simulink model "Tricopter_Controlled"  (R2015a)
settings: Solver=ode3  SolverMode=SingleTasking  StartTime=0.0  StopTime=inf  FixedStep=T_sim  RelTol=1e-3
values from neighbouring files (symbols this model uses):
  A_l_max_x = sqrt( (A_z_max)^2  -  g^2  )    [Run3Copter.m]
  A_l_max_y = g*tand(15)    [Run3Copter.m]
  A_z_max = Max_Thrust*3/m    [Run3Copter.m]
  Alt_0 = input(' Give the initial altitude (m): ')    [Run3Copter.m]
  B_hover_4dof = [-0.192641491537 -0.295051706147 -72.3190840892 -0.00308714144823 24.9504828653 -1.18743631629 9.87469464114e-05 6.48783896558 -0.0529805907426 -0.000387203135788 0.131620058452 2.24065603044 ... (54 elements, 6x9)]    [Effectiv_matrices.mat]
  CG_0 = [0,0,0.02]'    [SetupComplete.m]
  epsilon = 0.01    [Run3Copter.m]
  eta_23 = deg2rad(-1.3)    [Run3Copter.m]
  g = 9.81    [SetupComplete.m]
  h = 0.08    [SetupComplete.m]
  h_M = 0.064    [SetupComplete.m]
  Hover_eta_23 = deg2rad(-1.3)    [Run3Copter.m]
  Hover_throtle_1 = 0.745    [Run3Copter.m]
  Hover_throtle_23 = Hover_throtle_1/cos(Hover_eta_23)    [Run3Copter.m]
  I_BAC_0 = [ Ix,0,Ixz;0,Iy,0;Ixz,0,Iz]    [SetupComplete.m]
  Initial_Omegas = Omega_hover    [Run3Copter.m]
  Initial_Torques = Torque_hover    [Run3Copter.m]
  Ix = 0.103    [SetupComplete.m]
  Iy = 0.147    [SetupComplete.m]
  Iz = 0.237    [SetupComplete.m]
  l = 0.345    [SetupComplete.m]
  l_arm = 0.264    [SetupComplete.m]
  latitude = 52.071118    [Run3Copter.m]
  longitude = -0.627404    [Run3Copter.m]
  m = 3.51    [SetupComplete.m]
  m_0 = 2.61    [SetupComplete.m]
  m_M = 0.300    (= 0.3)    [SetupComplete.m]
  Rotation_sign = [ 1,-1,-1]    [SetupComplete.m]
  T_ctrl = 0.02    [Run3Copter.m]
  T_sim = 0.01    [Run3Copter.m]
  throtle_1 = 0*0.745    (= 0)    [Run3Copter.m]
  throtle_23 = throtle_1/cos(eta_23)    [Run3Copter.m]
  v_i0 = sqrt( 1/3*m*g/(2*rho*pi*R^2)  )    [SetupComplete.m]
undefined symbols (not defined in the file or in its folder): DOWN_0, EAST_0, Newton, NORTH_0, P_0, Q_0, R_0, Raphson, U_0, V_0, W_0
libraries: XXCopter_Control x64, simulink_extras x17, simulink x11, XXCopter x8
(part 2 of 6)

== system Tricopter_Controlled/Sensors and filtering. No noise/Sensors and filtering. No noise ==
  state : Inport
  Bus Creator : BusCreator  Inputs=9
  Bus Selector2 : BusSelector  OutputSignals=X_e,V_b,V_e,omega_b,q,euler,A_s
  Current batrery level (V) : Constant  Value=14.8
  Demux : Demux  Outputs=3
  Gain{1..7} (7 alike) : Gain
  Gain8 : Gain  Gain=-1
  Terminator : Terminator
  Terminator1 : Terminator
  keep -pi/pi1 : Subsystem
  All_measures : Outport
  wires:
  keep -pi/pi1/1(out (rad)) -> Gain2/1
  Gain6/1 -> Bus Creator/1  "Pos meas (m)"
  Gain5/1 -> Bus Creator/6  "q_meas"
  Bus Selector2/5 -> Gain5/1  "<q>"
  Gain4/1 -> Bus Creator/4  "V_e_meas"
  Bus Selector2/3 -> Gain4/1  "<V_e>"
  Gain1/1 -> Bus Creator/8  "A_accel meas"
  Bus Selector2/7 -> Gain1/1  "<A_s>"
  Gain2/1 -> Bus Creator/7  "Euler meas (rad)"
  Demux/3 -> Gain8/1  "Alt meas (m)"
  Bus Creator/1 -> All_measures/1
  Gain3/1 -> Bus Creator/5  "omega_b meas (rad/s)"
  Gain7/1 -> Bus Creator/3  "V_b_meas"
  Bus Selector2/6 -> keep -pi/pi1/1(in (rad))  "<euler>"
  Bus Selector2/4 -> Gain3/1  "<omega_b>"
  Bus Selector2/2 -> Gain7/1  "<V_b>"
  Demux/2 -> Terminator1/1
  Demux/1 -> Terminator/1
  Gain8/1 -> Bus Creator/2  "Alt meas (m)"
  Bus Selector2/1 -> Demux/1, Gain6/1  "<X_e>"
  state/1 -> Bus Selector2/1
  Current batrery level (V)/1 -> Bus Creator/9  "Volt"

== system Tricopter_Controlled/Sensors and filtering. No noise/Sensors and filtering. Noise ==
  note: Basado en https://pixhawk.org/firmware/parameters#attitude_ekf_estimator
  state : Inport
  Add{1..5} (5 alike) : Sum  Inputs=++|
  Add6 : Sum  Inputs=|++
  Add7 : Sum  Inputs=|++
  Add8 : Sum  Inputs=|++
  Bus Creator : BusCreator  Inputs=9
  Bus Selector2 : BusSelector  OutputSignals=X_e,V_b,V_e,omega_b,q,euler,A_s
  Current batrery level (V) : Constant  Value=14.8
  Demux : Demux  Outputs=[2,1]
  Gain{1..7} (7 alike) : Gain
  Gain14 : Gain  Gain=[1;1;1]
  Gain8 : Gain  Gain=-1
  Mux : Mux  Inputs=[2,1]
  Uniform Random Number : UniformRandomNumber  Minimum=-0.5*[1;1]  Maximum=0.5*[1;1]  Seed=[1,4]  SampleTime=T_sim*2
  Uniform Random Number1 : UniformRandomNumber  Minimum=-0.1  Maximum=0.1  Seed=3  SampleTime=T_sim*2  VectorParams1D=off
  Uniform Random Number2 : UniformRandomNumber  Minimum=-0.05  Maximum=0.05  Seed=[4,5,8]  SampleTime=T_sim*2
  Uniform Random Number3 : UniformRandomNumber  Minimum=-0.05  Maximum=0.05  Seed=[4,5,8]  SampleTime=T_sim*2
  Uniform Random Number4 : UniformRandomNumber  Minimum=-deg2rad(0.01)  Maximum=deg2rad(0.01)  Seed=[47,6,80]  SampleTime=T_sim*2
  Uniform Random Number5 : UniformRandomNumber  Minimum=-deg2rad(0.1/360)  Maximum=deg2rad(0.1/360)  Seed=[4,78,8,2]  SampleTime=T_sim*2
  Uniform Random Number6 : UniformRandomNumber  Minimum=-deg2rad(0.1)  Maximum=deg2rad(0.1)  Seed=[40,50,80]  SampleTime=T_sim*2
  Uniform Random Number7 : UniformRandomNumber  Minimum=-0.01*9.81  Maximum=0.01*9.81  Seed=[4,5,8]  SampleTime=T_sim*2
  keep -pi/pi1 : Subsystem
  All_measures : Outport
  wires:
  Gain6/1 -> Bus Creator/1  "Pos meas (m)"
  Gain5/1 -> Bus Creator/6  "q_meas"
  Add2/1 -> Gain5/1
  Gain4/1 -> Bus Creator/4  "V_e_meas"
  Add8/1 -> Gain4/1
  Gain1/1 -> Bus Creator/8  "A_accel meas(m/s^2)"
  Gain2/1 -> Bus Creator/7  "Euler meas (rad)"
  Bus Creator/1 -> All_measures/1
  Gain3/1 -> Bus Creator/5  "omega_b meas (rad/s)"
  Gain7/1 -> Bus Creator/3  "V_b_meas"
  Bus Selector2/6 -> keep -pi/pi1/1(in (rad))  "<euler>"
  Add4/1 -> Gain3/1
  Add7/1 -> Gain7/1
  Gain8/1 -> Bus Creator/2  "Alt meas (m)"
  Bus Selector2/1 -> Demux/1  "<X_e>"
  state/1 -> Bus Selector2/1
  Bus Selector2/5 -> Add2/2  "<q>"
  Add1/1 -> Gain2/1
  keep -pi/pi1/1(out (rad)) -> Gain14/1
  Add3/1 -> Gain1/1
  Bus Selector2/7 -> Add3/2  "<A_s>"
  Bus Selector2/4 -> Add4/2  "<omega_b>"
  Demux/1 -> Add5/2
  Add5/1 -> Mux/1
  Add6/1 -> Gain8/1, Mux/2
  Demux/2 -> Add6/1
  Mux/1 -> Gain6/1
  Uniform Random Number1/1 -> Add6/2
  Bus Selector2/2 -> Add7/1  "<V_b>"
  Bus Selector2/3 -> Add8/1  "<V_e>"
  Uniform Random Number/1 -> Add5/1
  Uniform Random Number2/1 -> Add7/2
  Uniform Random Number3/1 -> Add8/2
  Uniform Random Number4/1 -> Add4/1
  Uniform Random Number5/1 -> Add2/1
  Gain14/1 -> Add1/2
  Uniform Random Number7/1 -> Add3/1
  Uniform Random Number6/1 -> Add1/1
  Current batrery level (V)/1 -> Bus Creator/9  "Volt"

== system Tricopter_Controlled/Signals reality/PWM resolution ==
  PWM_us in : Inport
  Quantizer : Quantizer  QuantizationInterval=5
  PWM_us out : Outport
  wires:
  PWM_us in/1 -> Quantizer/1
  Quantizer/1 -> PWM_us out/1

== system Tricopter_Controlled/Signals reality/PWM resolution1 ==
  PWM_us in : Inport
  Quantizer : Quantizer  QuantizationInterval=5
  PWM_us out : Outport
  wires:
  Quantizer/1 -> PWM_us out/1
  PWM_us in/1 -> Quantizer/1

== system Tricopter_Controlled/Signals reality/Re-Build Signals servos ==
  note: Control input
      | Rango
      | Direccion rot/Dir servos
      | Rango del servo
      |
      | eta_1 (rad) (Pan arm 1)
      | -165,165
      | -1
      | 330: -165,165
      |
      | gamma_1 (rad) (Tilt arm 1)
      | -90,15
      | -1
      | 180:-90,90 ó 330: -165,165
      |
      | eta_2 (rad) (Pan arm 2)
      | -165,165
      | -1
      | 330: -165,165
      |
      | gamma_2 (rad) (Tilt arm 2)
      | -15,90
      | 1
      | 180:-90,90
      |
      | eta_3 (rad) (Pan arm 3)
      | -165,165
      | 1
      | 330:-165,165
      |
      | gamma_3 (rad) (Tilt arm 3)
      | -90,15
      | -1
      | 180:-90,90
  PWM_us servos in : Inport
  Demux : Demux  Outputs=6
  Mux : Mux  Inputs=6
  PWM2signal : XXCopter_Control/PWM2signal  c=2100  a=900  d=deg2rad(90)  b=-deg2rad(90)
  PWM2signal1 : XXCopter_Control/PWM2signal  c=2100  a=900  d=deg2rad(165)  b=-deg2rad(165)
  PWM2signal2 : XXCopter_Control/PWM2signal  c=2100  a=900  d=deg2rad(90)  b=-deg2rad(90)
  PWM2signal3 : XXCopter_Control/PWM2signal  c=2100  a=900  d=deg2rad(90)  b=-deg2rad(90)
  PWM2signal4 : XXCopter_Control/PWM2signal  c=2100  a=900  d=deg2rad(165)  b=-deg2rad(165)
  PWM2signal5 : XXCopter_Control/PWM2signal  c=2100  a=900  d=deg2rad(165)  b=-deg2rad(165)
  Unary Minus{,1..3} (4 alike) : UnaryMinus
  signals out : Outport
  wires:
  PWM_us servos in/1 -> Demux/1
  Demux/6 -> PWM2signal3/1
  Demux/5 -> PWM2signal5/1
  Demux/4 -> PWM2signal2/1
  Demux/3 -> PWM2signal4/1
  Demux/2 -> PWM2signal/1
  Demux/1 -> PWM2signal1/1
  PWM2signal1/1 -> Unary Minus/1
  PWM2signal/1 -> Unary Minus1/1
  PWM2signal4/1 -> Unary Minus2/1
  PWM2signal2/1 -> Mux/4
  PWM2signal5/1 -> Mux/5
  PWM2signal3/1 -> Unary Minus3/1
  Mux/1 -> signals out/1
  Unary Minus/1 -> Mux/1
  Unary Minus1/1 -> Mux/2
  Unary Minus2/1 -> Mux/3
  Unary Minus3/1 -> Mux/6

== system Tricopter_Controlled/TriCopter FCS/Interface out ==
  In1 : Inport
  In2 : Inport  Port=2
  In3 : Inport  Port=3
  In4 : Inport  Port=4
  In5 : Inport  Port=5
  In6 : Inport  Port=6
  In7 : Inport  Port=7
  In8 : Inport  Port=8
  In9 : Inport  Port=9
  Mux : Mux  Inputs=3
  Mux1 : Mux  Inputs=6
  Out1 : Outport
  Out2 : Outport  Port=2
  wires:
  Mux/1 -> Out1/1
  In1/1 -> Mux/1
  In4/1 -> Mux/2
  In7/1 -> Mux/3
  In2/1 -> Mux1/1
  In3/1 -> Mux1/2
  In5/1 -> Mux1/3
  In6/1 -> Mux1/4
  In8/1 -> Mux1/5
  In9/1 -> Mux1/6
  Mux1/1 -> Out2/1

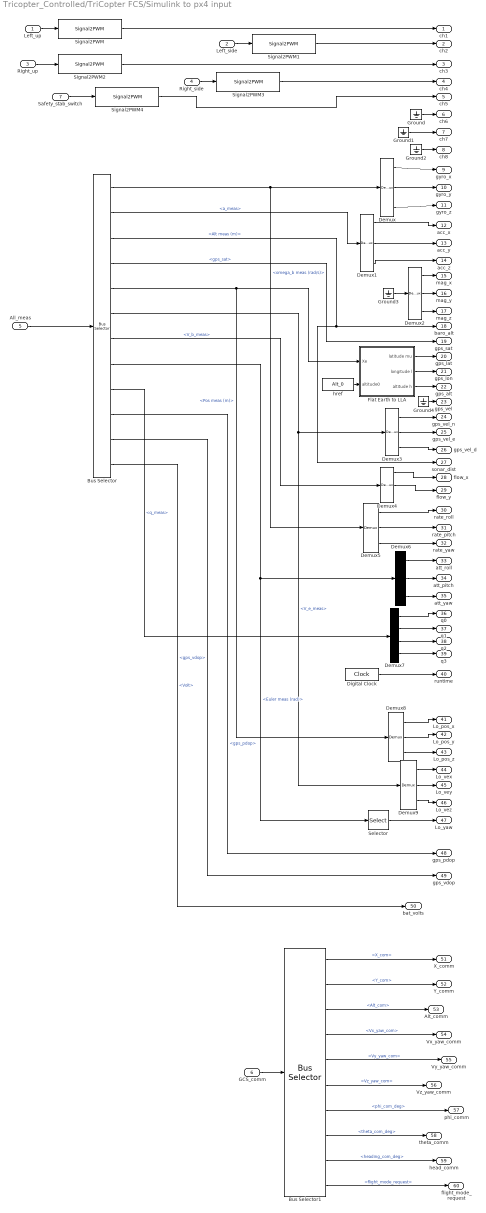
== system Tricopter_Controlled/TriCopter FCS/Simulink to px4 input ==
  Left_up : Inport
  Left_side : Inport  Port=2
  Right_up : Inport  Port=3
  Right_side : Inport  Port=4
  All_meas : Inport  Port=5
  GCS_comm : Inport  Port=6
  Safety_stab_switch : Inport  Port=7
  Bus Selector : BusSelector  OutputSignals=Meas.omega_b meas (rad/s),Params.a_meas,Meas.Alt meas (m),Params.gps_sat,Meas.Pos meas (m),Meas.V_e_meas,Meas.V_b_meas,Meas.Euler meas (rad),Meas.q_meas,Params.gps_pdop,Params.gps_vdop,Meas.Volt
  Bus Selector1 : BusSelector  OutputSignals=X_com,Y_com,Alt_com,Vx_yaw_com,Vy_yaw_com,Vz_yaw_com,phi_com_deg,theta_com_deg,heading_com_deg,flight_mode_request
  Demux{,1..6,8..9} (9 alike) : Demux  Outputs=3
  Demux7 : Demux
  Digital Clock : DigitalClock  SampleTime=T_ctrl
  Flat Earth to LLA : Subsystem
  Ground{,1..4} (5 alike) : Ground
  Selector : Selector  InputPortWidth=3  Indices=3
  Signal2PWM{,1..3} (4 alike) : XXCopter_Control/Signal2PWM  b=1  d=-1  a=1800  c=1200
  Signal2PWM4 : XXCopter_Control/Signal2PWM  b=1  d=0  a=1800  c=1200
  href : Constant  Value=Alt_0  VectorParams1D=off
  ch1 : Outport
  ch2 : Outport  Port=2
  ch3 : Outport  Port=3
  ch4 : Outport  Port=4
  ch5 : Outport  Port=5
  ch6 : Outport  Port=6
  ch7 : Outport  Port=7
  ch8 : Outport  Port=8
  gyro_x : Outport  Port=9
  gyro_y : Outport  Port=10
  gyro_z : Outport  Port=11
  acc_x : Outport  Port=12
  acc_y : Outport  Port=13
  acc_z : Outport  Port=14
  mag_x : Outport  Port=15
  mag_y : Outport  Port=16
  mag_z : Outport  Port=17
  baro_alt : Outport  Port=18
  gps_sat : Outport  Port=19
  gps_lat : Outport  Port=20
  gps_lon : Outport  Port=21
  gps_alt : Outport  Port=22
  gps_vel : Outport  Port=23
  gps_vel_n : Outport  Port=24
  gps_vel_e : Outport  Port=25
  gps_vel_d : Outport  Port=26
  sonar_dist : Outport  Port=27
  flow_x : Outport  Port=28
  flow_y : Outport  Port=29
  rate_roll : Outport  Port=30
  rate_pitch : Outport  Port=31
  rate_yaw : Outport  Port=32
  att_roll : Outport  Port=33
  att_pitch : Outport  Port=34
  att_yaw : Outport  Port=35
  q0 : Outport  Port=36
  q1 : Outport  Port=37
  q2 : Outport  Port=38
  q3 : Outport  Port=39
  runtime : Outport  Port=40
  Lo_pos_x : Outport  Port=41
  Lo_pos_y : Outport  Port=42
  Lo_pos_z : Outport  Port=43
  Lo_vex : Outport  Port=44
  Lo_vey : Outport  Port=45
  Lo_vez : Outport  Port=46
  Lo_yaw : Outport  Port=47
  gps_pdop : Outport  Port=48
  gps_vdop : Outport  Port=49
  bat_volts : Outport  Port=50
  X_comm : Outport  Port=51
  Y_comm : Outport  Port=52
  Alt_comm : Outport  Port=53
  Vx_yaw_comm : Outport  Port=54
  Vy_yaw_comm : Outport  Port=55
  Vz_yaw_comm : Outport  Port=56
  phi_comm : Outport  Port=57
  theta_comm : Outport  Port=58
  head_comm : Outport  Port=59
  flight_mode_request : Outport  Port=60
  wires:
  Left_up/1 -> Signal2PWM/1
  Left_side/1 -> Signal2PWM1/1
  Right_up/1 -> Signal2PWM2/1
  Right_side/1 -> Signal2PWM3/1
  Safety_stab_switch/1 -> Signal2PWM4/1
  Ground/1 -> ch6/1
  Ground1/1 -> ch7/1
  Ground2/1 -> ch8/1
  All_meas/1 -> Bus Selector/1
  href/1 -> Flat Earth to LLA/2(altitude0)
  Demux/1 -> gyro_x/1
  Demux/2 -> gyro_y/1
  Demux/3 -> gyro_z/1
  Bus Selector/1 -> Demux5/1, Demux/1  "<omega_b meas (rad/s)>"
  Demux1/1 -> acc_x/1
  Demux1/2 -> acc_y/1
  Demux1/3 -> acc_z/1
  Bus Selector/2 -> Demux1/1  "<a_meas>"
  Ground3/1 -> Demux2/1
  Demux2/1 -> mag_x/1
  Demux2/2 -> mag_y/1
  Demux2/3 -> mag_z/1
  Bus Selector/3 -> baro_alt/1, sonar_dist/1  "<Alt meas (m)>"
  Bus Selector/4 -> gps_sat/1  "<gps_sat>"
  Flat Earth to LLA/1(latitude mu) -> gps_lat/1
  Flat Earth to LLA/2(longitude l) -> gps_lon/1
  Flat Earth to LLA/3(altitude h) -> gps_alt/1
  Bus Selector/5 -> Flat Earth to LLA/1(Xe), Demux8/1  "<Pos meas (m)>"
  Ground4/1 -> gps_vel/1
  Demux3/1 -> gps_vel_n/1
  Demux3/3 -> gps_vel_d/1
  Bus Selector/6 -> Demux9/1, Demux3/1  "<V_e_meas>"
  Demux3/2 -> gps_vel_e/1
  Bus Selector/7 -> Demux4/1  "<V_b_meas>"
  Demux4/2 -> flow_y/1
  Demux4/1 -> flow_x/1
  Demux5/1 -> rate_roll/1
  Demux5/2 -> rate_pitch/1
  Demux5/3 -> rate_yaw/1
  Demux6/1 -> att_roll/1
  Demux6/2 -> att_pitch/1
  Demux6/3 -> att_yaw/1
  Bus Selector/8 -> Selector/1, Demux6/1  "<Euler meas (rad)>"
  Demux7/1 -> q0/1
  Demux7/2 -> q1/1
  Demux7/3 -> q2/1
  Demux7/4 -> q3/1
  Bus Selector/9 -> Demux7/1  "<q_meas>"
  Demux8/1 -> Lo_pos_x/1
  Demux8/2 -> Lo_pos_y/1
  Demux8/3 -> Lo_pos_z/1
  Demux9/1 -> Lo_vex/1
  Demux9/2 -> Lo_vey/1
  Demux9/3 -> Lo_vez/1
  Selector/1 -> Lo_yaw/1
  Bus Selector/10 -> gps_pdop/1  "<gps_pdop>"
  Bus Selector/11 -> gps_vdop/1  "<gps_vdop>"
  Bus Selector/12 -> bat_volts/1  "<Volt>"
  GCS_comm/1 -> Bus Selector1/1
  Bus Selector1/1 -> X_comm/1  "<X_com>"
  Bus Selector1/2 -> Y_comm/1  "<Y_com>"
  Bus Selector1/3 -> Alt_comm/1  "<Alt_com>"
  Bus Selector1/4 -> Vx_yaw_comm/1  "<Vx_yaw_com>"
  Bus Selector1/5 -> Vy_yaw_comm/1  "<Vy_yaw_com>"
  Bus Selector1/6 -> Vz_yaw_comm/1  "<Vz_yaw_com>"
  Bus Selector1/7 -> phi_comm/1  "<phi_com_deg>"
  Bus Selector1/8 -> theta_comm/1  "<theta_com_deg>"
  Bus Selector1/9 -> head_comm/1  "<heading_com_deg>"
  Bus Selector1/10 -> flight_mode_request/1  "<flight_mode_request>"
  Signal2PWM/1 -> ch1/1
  Signal2PWM1/1 -> ch2/1
  Signal2PWM2/1 -> ch3/1
  Signal2PWM3/1 -> ch4/1
  Signal2PWM4/1 -> ch5/1
  Digital Clock/1 -> runtime/1

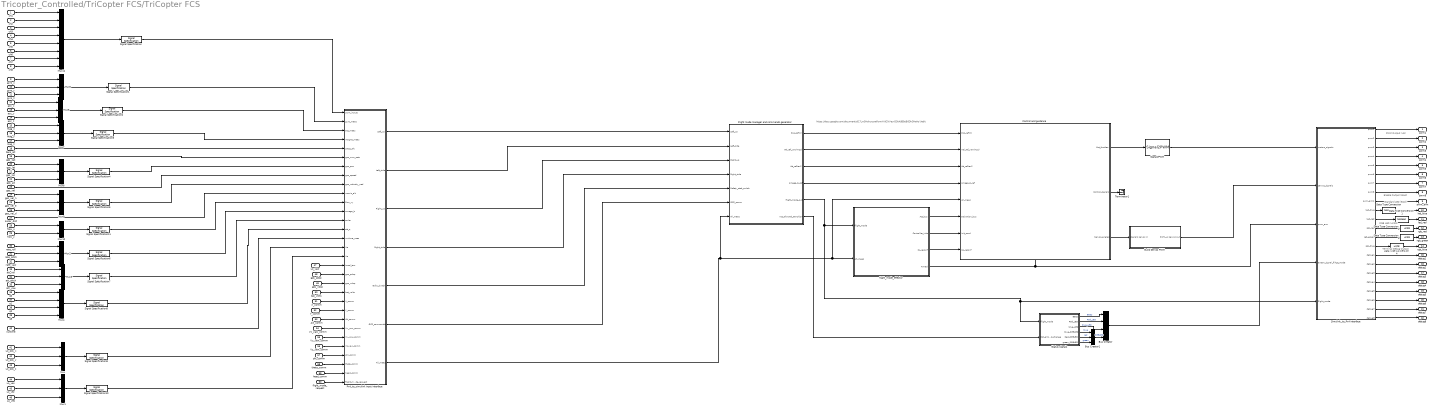
== system Tricopter_Controlled/TriCopter FCS/TriCopter FCS ==
  note: https://docs.google.com/document/d/17Lw5HdxcxpxePsmAYdCNVeyrDDt4j9EbtB6DkGHaHsY/edit
  note: Terminal Debug Output
  note: RGB LED (uint8)
  note: Standard LED (Bool)
  note: PWM Output (uS)
  note: Enable Output (Bool)
  ch1 : Inport  PortDimensions=[1,1]  SampleTime=T_ctrl
  ch2 : Inport  Port=2  PortDimensions=[1,1]  SampleTime=T_ctrl
  ch3 : Inport  Port=3  PortDimensions=[1,1]  SampleTime=T_ctrl
  ch4 : Inport  Port=4  PortDimensions=[1,1]  SampleTime=T_ctrl
  ch5 : Inport  Port=5  PortDimensions=[1,1]  SampleTime=T_ctrl
  ch6 : Inport  Port=6  PortDimensions=[1,1]  SampleTime=T_ctrl
  ch7 : Inport  Port=7  PortDimensions=[1,1]  SampleTime=T_ctrl
  ch8 : Inport  Port=8  PortDimensions=[1,1]  SampleTime=T_ctrl
  gyro_x : Inport  Port=9  PortDimensions=[1,1]  SampleTime=T_ctrl
  gyro_y : Inport  Port=10  PortDimensions=[1,1]  SampleTime=T_ctrl
  gyro_z : Inport  Port=11  PortDimensions=[1,1]  SampleTime=T_ctrl
  acc_x : Inport  Port=12  PortDimensions=[1,1]  SampleTime=T_ctrl
  acc_y : Inport  Port=13  PortDimensions=[1,1]  SampleTime=T_ctrl
  acc_z : Inport  Port=14  PortDimensions=[1,1]  SampleTime=T_ctrl
  mag_x : Inport  Port=15  PortDimensions=[1,1]  SampleTime=T_ctrl
  mag_y : Inport  Port=16  PortDimensions=[1,1]  SampleTime=T_ctrl
  mag_z : Inport  Port=17  PortDimensions=[1,1]  SampleTime=T_ctrl
  baro_alt : Inport  Port=18  PortDimensions=[1,1]  SampleTime=T_ctrl
  gps_sat : Inport  Port=19  PortDimensions=[1,1]  SampleTime=T_ctrl
  gps_lat : Inport  Port=20  PortDimensions=[1,1]  SampleTime=T_ctrl
  gps_lon : Inport  Port=21  PortDimensions=[1,1]  SampleTime=T_ctrl
  gps_alt : Inport  Port=22  PortDimensions=[1,1]  SampleTime=T_ctrl
  gps_vel : Inport  Port=23  PortDimensions=[1,1]  SampleTime=T_ctrl
  gps_vel_n : Inport  Port=24  PortDimensions=[1,1]  SampleTime=T_ctrl
  gps_vel_e : Inport  Port=25  PortDimensions=[1,1]  SampleTime=T_ctrl
  gps_vel_d : Inport  Port=26  PortDimensions=[1,1]  SampleTime=T_ctrl
  sonar_dist : Inport  Port=27  PortDimensions=[1,1]  SampleTime=T_ctrl
  flow_x : Inport  Port=28  PortDimensions=[1,1]  SampleTime=T_ctrl
  flow_y : Inport  Port=29  PortDimensions=[1,1]  SampleTime=T_ctrl
  rate_roll : Inport  Port=30  PortDimensions=[1,1]  SampleTime=T_ctrl
  rate_pitch : Inport  Port=31  PortDimensions=[1,1]  SampleTime=T_ctrl
  rate_yaw : Inport  Port=32  PortDimensions=[1,1]  SampleTime=T_ctrl
  att_roll : Inport  Port=33  PortDimensions=[1,1]  SampleTime=T_ctrl
  att_pitch : Inport  Port=34  PortDimensions=[1,1]  SampleTime=T_ctrl
  att_yaw : Inport  Port=35  PortDimensions=[1,1]  SampleTime=T_ctrl
  q0 : Inport  Port=36  PortDimensions=[1,1]  SampleTime=T_ctrl
  q1 : Inport  Port=37  PortDimensions=[1,1]  SampleTime=T_ctrl
  q2 : Inport  Port=38  PortDimensions=[1,1]  SampleTime=T_ctrl
  q3 : Inport  Port=39  PortDimensions=[1,1]  SampleTime=T_ctrl
  runtime : Inport  Port=40  PortDimensions=[1,1]  SampleTime=T_ctrl
  Lo_pos_x : Inport  Port=41  PortDimensions=[1,1]  SampleTime=T_ctrl
  Lo_pos_y : Inport  Port=42  PortDimensions=[1,1]  SampleTime=T_ctrl
  Lo_pos_z : Inport  Port=43  PortDimensions=[1,1]  SampleTime=T_ctrl
  Lo_vex : Inport  Port=44  PortDimensions=[1,1]  SampleTime=T_ctrl
  Lo_vey : Inport  Port=45  PortDimensions=[1,1]  SampleTime=T_ctrl
  Lo_vez : Inport  Port=46  PortDimensions=[1,1]  SampleTime=T_ctrl
  Lo_yaw : Inport  Port=47  PortDimensions=[1,1]  SampleTime=T_ctrl
  gps_pdop : Inport  Port=48  PortDimensions=[1,1]  SampleTime=T_ctrl
  gps_vdop : Inport  Port=49  PortDimensions=[1,1]  SampleTime=T_ctrl
  bat_volts : Inport  Port=50  PortDimensions=[1,1]  SampleTime=T_ctrl
  X_comm : Inport  Port=51  PortDimensions=[1,1]  SampleTime=T_ctrl
  Y_comm : Inport  Port=52  PortDimensions=[1,1]  SampleTime=T_ctrl
  Alt_comm : Inport  Port=53  PortDimensions=[1,1]  SampleTime=T_ctrl
  Vx_yaw_comm : Inport  Port=54  PortDimensions=[1,1]  SampleTime=T_ctrl
  Vy_yaw_comm : Inport  Port=55  PortDimensions=[1,1]  SampleTime=T_ctrl
  Vz_yaw_comm : Inport  Port=56  PortDimensions=[1,1]  SampleTime=T_ctrl
  phi_comm : Inport  Port=57  PortDimensions=[1,1]  SampleTime=T_ctrl
  theta_comm : Inport  Port=58  PortDimensions=[1,1]  SampleTime=T_ctrl
  head_comm : Inport  Port=59  PortDimensions=[1,1]  SampleTime=T_ctrl
  flight_mode_request : Inport  Port=60  PortDimensions=[1,1]  SampleTime=T_ctrl
  Build Servos PWM : Subsystem  TreatAsAtomicUnit=on
  Bus Creator : BusCreator
  Bus Creator1 : BusCreator  Inputs=3
  Control and guidance : Subsystem
  Data Type Conversion : DataTypeConversion  OutDataTypeStr=boolean
  Data Type Conversion1 : DataTypeConversion  OutDataTypeStr=boolean
  Data Type Conversion2 : DataTypeConversion  OutDataTypeStr=uint8
  Data Type Conversion3 : DataTypeConversion  OutDataTypeStr=uint8
  Data Type Conversion4 : DataTypeConversion  OutDataTypeStr=uint8
  Flight mode manager and commands generator : Subsystem
  Mux{,1..3,5..9} (9 alike) : Mux  Inputs=3
  Mux10 : Mux  Inputs=2
  Mux11 : Mux  Inputs=8
  Mux4 : Mux
  Px4_to_simulink input interface : Subsystem
  Signal Specification : SignalSpecification  Dimensions=[8,1]
  Signal Specification{1..7,9..10} (9 alike) : SignalSpecification  Dimensions=[3,1]
  Signal Specification11 : SignalSpecification  Dimensions=[2,1]
  Signal Specification8 : SignalSpecification  Dimensions=[4,1]
  Signal2PWM : XXCopter_Control/Signal2PWM  b=1  d=0  a=1800  c=1200
  Simulink_to_Px4 interface : Subsystem
  Status signals : Subsystem  TreatAsAtomicUnit=on
  Terminator1 : Terminator
  flight_mode_effector : Subsystem
  pwm1 : Outport  PortDimensions=[1,1]
  pwm2 : Outport  Port=2  PortDimensions=[1,1]
  pwm3 : Outport  Port=3  PortDimensions=[1,1]
  pwm4 : Outport  Port=4  PortDimensions=[1,1]
  pwm5 : Outport  Port=5  PortDimensions=[1,1]
  pwm6 : Outport  Port=6  PortDimensions=[1,1]
  pwm7 : Outport  Port=7  PortDimensions=[1,1]
  pwm8 : Outport  Port=8  PortDimensions=[1,1]
  pwm_arm : Outport  Port=9  PortDimensions=[1,1]
  led_blue : Outport  Port=10  OutDataTypeStr=boolean  PortDimensions=[1,1]
  led_red : Outport  Port=11  OutDataTypeStr=boolean  PortDimensions=[1,1]
  rgb_red : Outport  Port=12  OutDataTypeStr=uint8  PortDimensions=[1,1]
  rgb_green : Outport  Port=13  OutDataTypeStr=uint8  PortDimensions=[1,1]
  rgb_blue : Outport  Port=14  OutDataTypeStr=uint8  PortDimensions=[1,1]
  debug1 : Outport  Port=15  PortDimensions=[1,1]
  debug2 : Outport  Port=16  PortDimensions=[1,1]
  debug3 : Outport  Port=17  PortDimensions=[1,1]
  debug4 : Outport  Port=18  PortDimensions=[1,1]
  debug5 : Outport  Port=19  PortDimensions=[1,1]
  debug6 : Outport  Port=20  PortDimensions=[1,1]
  debug7 : Outport  Port=21  PortDimensions=[1,1]
  debug8 : Outport  Port=22  PortDimensions=[1,1]
  wires:
  Flight mode manager and commands generator/1(Pos_ref(m)) -> Control and guidance/1(Pos_ref(m))
  Flight mode manager and commands generator/2(Vel_ref_yaw(mps)) -> Control and guidance/2(Vel_ref_yaw(mps))
  Flight mode manager and commands generator/3(Att_ref(rad)) -> Control and guidance/3(Att_ref(rad))
  Control and guidance/1(Mot_throtles) -> Signal2PWM/1
  Control and guidance/3(Servos_angles) -> Build Servos PWM/1(signals servos in)
  Flight mode manager and commands generator/4(omega_b_ref) -> Control and guidance/4(omega_b_ref)
  flight_mode_effector/1(Act_bus) -> Control and guidance/6(activation_bus)
  flight_mode_effector/2(Controller_inits) -> Control and guidance/7(Init_cond)
  flight_mode_effector/3(CA_reconf) -> Control and guidance/8(CA_reconf)
  Flight mode manager and commands generator/6(not_allowed_transition) -> Status signals/2(Not_allowed_change)
  Status signals/1(Beep) -> Bus Creator/1  "Beep"
  Status signals/2(Red_LED) -> Bus Creator/2  "Red_LED"
  Status signals/3(blue_LED) -> Bus Creator/3  "blue_LED"
  Status signals/4(blue_RGBLED) -> Bus Creator1/1  "blue"
  Status signals/5(Red_RGBLED) -> Bus Creator1/2  "red"
  Status signals/6(green_RGBLED) -> Bus Creator1/3  "green"
  Bus Creator1/1 -> Bus Creator/4  "RGBLED"
  Simulink_to_Px4 interface/1(pwm1) -> pwm1/1
  Simulink_to_Px4 interface/2(pwm2) -> pwm2/1
  Simulink_to_Px4 interface/3(pwm3) -> pwm3/1
  Simulink_to_Px4 interface/4(pwm4) -> pwm4/1
  Simulink_to_Px4 interface/5(pwm5) -> pwm5/1
  Simulink_to_Px4 interface/6(pwm6) -> pwm6/1
  Simulink_to_Px4 interface/7(pwm7) -> pwm7/1
  Simulink_to_Px4 interface/8(pwm8) -> pwm8/1
  Simulink_to_Px4 interface/10(led_blue) -> Data Type Conversion/1
  Simulink_to_Px4 interface/11(led_red) -> Data Type Conversion1/1
  Simulink_to_Px4 interface/15(debug1) -> debug1/1
  Simulink_to_Px4 interface/17(debug3) -> debug3/1
  Simulink_to_Px4 interface/18(debug4) -> debug4/1
  Simulink_to_Px4 interface/9(pwm_arm1) -> pwm_arm/1
  Simulink_to_Px4 interface/12(rgb_red) -> Data Type Conversion2/1
  Simulink_to_Px4 interface/13(rgb_green) -> Data Type Conversion3/1
  Simulink_to_Px4 interface/14(rgb_blue) -> Data Type Conversion4/1
  Simulink_to_Px4 interface/20(debug6) -> debug6/1
  Simulink_to_Px4 interface/21(debug7) -> debug7/1
  Simulink_to_Px4 interface/22(debug8) -> debug8/1
  Simulink_to_Px4 interface/19(debug5) -> debug5/1
  flight_mode_effector/4(Armed) -> Simulink_to_Px4 interface/3(pwm_arm), Control and guidance/Enable
  Data Type Conversion/1 -> led_blue/1
  Data Type Conversion1/1 -> led_red/1
  Flight mode manager and commands generator/5(flight_mode_out) -> Simulink_to_Px4 interface/5(flight_mode), Status signals/1(flight_mode), flight_mode_effector/1(flight_mode)
  Data Type Conversion2/1 -> rgb_red/1
  Data Type Conversion3/1 -> rgb_green/1
  Data Type Conversion4/1 -> rgb_blue/1
  Control and guidance/2(Control_signals) -> Terminator1/1
  Simulink_to_Px4 interface/16(debug2) -> debug2/1
  Signal2PWM/1 -> Simulink_to_Px4 interface/1(motors_signals)
  Build Servos PWM/1(PWM_us servos out) -> Simulink_to_Px4 interface/2(servos_signals)
  Bus Creator/1 -> Simulink_to_Px4 interface/4(extern_signal_flihgt_mode)
  Px4_to_simulink input interface/7(All_meas) -> Flight mode manager and commands generator/7(All_meas), Control and guidance/5(All_meas), flight_mode_effector/2(All_meas)
  sonar_dist/1 -> Px4_to_simulink input interface/10(usonic_alt)
  baro_alt/1 -> Px4_to_simulink input interface/5(press_alt)
  gyro_z/1 -> Mux6/3
  gyro_y/1 -> Mux6/2
  gyro_x/1 -> Mux6/1
  acc_z/1 -> Mux5/3
  acc_y/1 -> Mux5/2
  acc_x/1 -> Mux5/1
  mag_x/1 -> Mux7/1
  mag_y/1 -> Mux7/2
  mag_z/1 -> Mux7/3
  ch1/1 -> Mux11/1
  ch2/1 -> Mux11/2
  ch3/1 -> Mux11/3
  ch4/1 -> Mux11/4
  ch5/1 -> Mux11/5
  ch6/1 -> Mux11/6
  flow_y/1 -> Mux10/2
  flow_x/1 -> Mux10/1
  runtime/1 -> Px4_to_simulink input interface/15(runtime_usec)
  ch7/1 -> Mux11/7
  ch8/1 -> Mux11/8
  att_roll/1 -> Mux3/1
  att_pitch/1 -> Mux3/2
  att_yaw/1 -> Mux3/3
  q0/1 -> Mux4/1
  q1/1 -> Mux4/2
  q2/1 -> Mux4/3
  q3/1 -> Mux4/4
  rate_roll/1 -> Mux2/1
  rate_pitch/1 -> Mux2/2
  rate_yaw/1 -> Mux2/3
  gps_vel_n/1 -> Mux9/1
  gps_vel_e/1 -> Mux9/2
  gps_vel_d/1 -> Mux9/3
  gps_lat/1 -> Mux8/1
  gps_lon/1 -> Mux8/2
  gps_alt/1 -> Mux8/3
  gps_vel/1 -> Px4_to_simulink input interface/8(gps_speed)
  gps_sat/1 -> Px4_to_simulink input interface/6(gps_num_sats)
  Lo_pos_x/1 -> Mux/1
  Lo_pos_y/1 -> Mux/2
  Lo_pos_z/1 -> Mux/3
  Mux/1 -> Signal Specification9/1
  Lo_vex/1 -> Mux1/1
  Lo_vey/1 -> Mux1/2
  Lo_vez/1 -> Mux1/3
  Mux1/1 -> Signal Specification10/1
  Mux2/1 -> Signal Specification6/1
  Mux3/1 -> Signal Specification7/1
  Mux4/1 -> Signal Specification8/1
  Mux5/1 -> Signal Specification2/1
  Y_comm/1 -> Px4_to_simulink input interface/23(Y_comm)
  Alt_comm/1 -> Px4_to_simulink input interface/24(Alt_comm)
  Vx_yaw_comm/1 -> Px4_to_simulink input interface/25(Vx_yaw_comm)
  Vy_yaw_comm/1 -> Px4_to_simulink input interface/26(Vy_yaw_comm)
  theta_comm/1 -> Px4_to_simulink input interface/29(theta_comm)
  head_comm/1 -> Px4_to_simulink input interface/30(head_comm)
  flight_mode_request/1 -> Px4_to_simulink input interface/31(flight_mode_request)
  Mux6/1 -> Signal Specification1/1
  Mux8/1 -> Signal Specification4/1
  Mux7/1 -> Signal Specification3/1
  Mux11/1 -> Signal Specification/1
  Mux10/1 -> Signal Specification11/1
  Mux9/1 -> Signal Specification5/1
  Lo_yaw/1 -> Px4_to_simulink input interface/18(Local_taw)
  gps_pdop/1 -> Px4_to_simulink input interface/19(gps_pdop)
  gps_vdop/1 -> Px4_to_simulink input interface/20(gps_vdop)
  bat_volts/1 -> Px4_to_simulink input interface/21(bat_volts)
  X_comm/1 -> Px4_to_simulink input interface/22(X_comm)
  Vz_yaw_comm/1 -> Px4_to_simulink input interface/27(Vz_yaw_comm)
  phi_comm/1 -> Px4_to_simulink input interface/28(phi_comm)
  Px4_to_simulink input interface/1(Left_up) -> Flight mode manager and commands generator/1(Left_up)
  Px4_to_simulink input interface/2(Left_side) -> Flight mode manager and commands generator/2(Left_side)
  Px4_to_simulink input interface/3(Right_up) -> Flight mode manager and commands generator/3(Right_up)
  Px4_to_simulink input interface/4(Right_side) -> Flight mode manager and commands generator/4(Right_side)
  Px4_to_simulink input interface/5(radio_siwtch) -> Flight mode manager and commands generator/5(Safety_stab_switch)
  Px4_to_simulink input interface/6(GCS_commands) -> Flight mode manager and commands generator/6(GCS_comm)
  Signal Specification/1 -> Px4_to_simulink input interface/1(pwm_inputs)
  Signal Specification1/1 -> Px4_to_simulink input interface/2(gyro_meas)
  Signal Specification2/1 -> Px4_to_simulink input interface/3(acc_meas)
  Signal Specification3/1 -> Px4_to_simulink input interface/4(magne_meas)
  Signal Specification4/1 -> Px4_to_simulink input interface/7(gps_pos)
  Signal Specification5/1 -> Px4_to_simulink input interface/9(gps_velocity_ned)
  Signal Specification6/1 -> Px4_to_simulink input interface/12(omega_b)
  Signal Specification7/1 -> Px4_to_simulink input interface/13(euler)
  Signal Specification8/1 -> Px4_to_simulink input interface/14(att_q)
  Signal Specification9/1 -> Px4_to_simulink input interface/16(Xe)
  Signal Specification10/1 -> Px4_to_simulink input interface/17(Ve)
  Signal Specification11/1 -> Px4_to_simulink input interface/11(flow_xy)

== system Tricopter_Controlled/3 Copter Complete/6dof Eqs of motion/DCM1 ==
  Euler : Inport  PortDimensions=3
  Fcn11 : Fcn  Expr=u(5)*u(4)
  Fcn12 : Fcn  Expr=u(5)*u(1)
  Fcn13 : Fcn  Expr=-u(2)
  Fcn21 : Fcn  Expr=u(3)*u(2)*u(4) - u(6)*u(1)
  Fcn22 : Fcn  Expr=u(3)*u(2)*u(1) + u(6)*u(4)
  Fcn23 : Fcn  Expr=u(3)*u(5)
  Fcn31 : Fcn  Expr=u(6)*u(2)*u(4) + u(3)*u(1)
  Fcn32 : Fcn  Expr=u(6)*u(2)*u(1) - u(3)*u(4)
  Fcn33 : Fcn  Expr=u(6)*u(5)
  Mux : Mux  Inputs=2
  Mux1 : Mux  Inputs=9
  Reshape : Reshape  OutputDimensionality=Customize  OutputDimensions=[3,3]
  sincos : Trigonometry  Operator=sincos
  DCM : Outport  PortDimensions=[3,3]
  wires:
  Fcn33/1 -> Mux1/9
  Fcn32/1 -> Mux1/8
  Fcn23/1 -> Mux1/6
  Fcn22/1 -> Mux1/5
  Fcn31/1 -> Mux1/7
  Fcn21/1 -> Mux1/4
  Fcn13/1 -> Mux1/3
  Fcn12/1 -> Mux1/2
  Fcn11/1 -> Mux1/1
  Mux/1 -> Fcn22/1, Fcn23/1, Fcn31/1, Fcn33/1, Fcn32/1, Fcn21/1, Fcn13/1, Fcn12/1, Fcn11/1
  sincos/2 -> Mux/2
  sincos/1 -> Mux/1
  Reshape/1 -> DCM/1
  Euler/1 -> sincos/1
  Mux1/1 -> Reshape/1

== system Tricopter_Controlled/3 Copter Complete/6dof Eqs of motion/q_dot ==
  note: Both of these methods to compute q_dot are very similar
  omega_b : Inport
  q : Inport  Port=2
  Quaternion_dot : MATLAB Function  TreatAsAtomicUnit=on  VariantControl=Variant
  q_dot : Outport
  wires:
  omega_b/1 -> Quaternion_dot/1(omega_b)  "omega_b"
  q/1 -> Quaternion_dot/2(q)  "q"
  Quaternion_dot/1(q_dot) -> q_dot/1

== system Tricopter_Controlled/FlightGear visualization/Flat Earth to LLA/ne to lat//long ==
  Xe : Inport
  Demux : Demux  Outputs=2
  "Latitude Between +/- 90 " : Subsystem  TreatAsAtomicUnit=on
  "LongLat_offset " : Subsystem  TreatAsAtomicUnit=on
  "Longitude Between +/-180 " : Subsystem  TreatAsAtomicUnit=on
  Sel1 : Selector  InputPortWidth=3  Indices=[1,2]
  Sum2 : Sum  Inputs=++|
  initial_latg : Constant  Value=latitude
  initial_pos : Constant  Value=[latitude,longitude]
  rad2deg : Gain  Gain=180/pi  SaturateOnIntegerOverflow=on  OutDataTypeStr=Inherit: Same as input  ParamDataTypeStr=Inherit: Same as input
  lat_deg : Outport
  long_deg : Outport  Port=2
  wires:
  Xe/1 -> Sel1/1
  Sum2/1 -> "Latitude Between +/- 90 "/1(mu l)
  "LongLat_offset "/1(DeltaLL_rad) -> rad2deg/1
  Sel1/1 -> "LongLat_offset "/1(XY)
  rad2deg/1 -> Sum2/2
  initial_pos/1 -> Sum2/1
  initial_latg/1 -> "LongLat_offset "/2(mu)
  "Latitude Between +/- 90 "/1("mu l ") -> "Longitude Between +/-180 "/1(mu l)
  "Longitude Between +/-180 "/1("mu l ") -> Demux/1
  Demux/1 -> lat_deg/1
  Demux/2 -> long_deg/1

== system Tricopter_Controlled/Sensors and filtering. No noise/Sensors and filtering. No noise/keep -pi//pi1 ==
  in (rad) : Inport
  Constant : Constant  Value=180
  Constant2 : Constant  Value=360
  Gain : Gain  Gain=360
  Math Function2 : Math  Operator=rem  SaturateOnIntegerOverflow=on
  Product : Product  Inputs=*/  RndMeth=Zero
  Rounding Function : Rounding  Operator=fix
  Sum2 : Sum  Inputs=|-+
  deg2rad1 : Gain  Gain=pi/180  SaturateOnIntegerOverflow=on  OutDataTypeStr=Inherit: Same as input  ParamDataTypeStr=Inherit: Same as input
  rad2deg : Gain  Gain=180/pi  SaturateOnIntegerOverflow=on  OutDataTypeStr=Inherit: Same as input  ParamDataTypeStr=Inherit: Same as input
  out (rad) : Outport
  wires:
  deg2rad1/1 -> out (rad)/1
  Sum2/1 -> deg2rad1/1
  Math Function2/1 -> Sum2/2, Product/1
  Constant2/1 -> Math Function2/2
  rad2deg/1 -> Math Function2/1
  Gain/1 -> Sum2/1
  Rounding Function/1 -> Gain/1
  Product/1 -> Rounding Function/1
  Constant/1 -> Product/2
  in (rad)/1 -> rad2deg/1

== system Tricopter_Controlled/Sensors and filtering. No noise/Sensors and filtering. Noise/keep -pi//pi1 ==
  in (rad) : Inport
  Constant : Constant  Value=180
  Constant2 : Constant  Value=360
  Gain : Gain  Gain=360
  Math Function2 : Math  Operator=rem  SaturateOnIntegerOverflow=on
  Product : Product  Inputs=*/  RndMeth=Zero
  Rounding Function : Rounding  Operator=fix
  Sum2 : Sum  Inputs=|-+
  deg2rad1 : Gain  Gain=pi/180  SaturateOnIntegerOverflow=on  OutDataTypeStr=Inherit: Same as input  ParamDataTypeStr=Inherit: Same as input
  rad2deg : Gain  Gain=180/pi  SaturateOnIntegerOverflow=on  OutDataTypeStr=Inherit: Same as input  ParamDataTypeStr=Inherit: Same as input
  out (rad) : Outport
  wires:
  deg2rad1/1 -> out (rad)/1
  Sum2/1 -> deg2rad1/1
  Math Function2/1 -> Sum2/2, Product/1
  Constant2/1 -> Math Function2/2
  rad2deg/1 -> Math Function2/1
  Gain/1 -> Sum2/1
  Rounding Function/1 -> Gain/1
  Product/1 -> Rounding Function/1
  Constant/1 -> Product/2
  in (rad)/1 -> rad2deg/1

== system Tricopter_Controlled/TriCopter FCS/Simulink to px4 input/Flat Earth to LLA ==
  note: Flat Earth to LLA
  Xe : Inport
  altitude0 : Inport  Port=2
  Add : Sum
  Demux1 : Demux  Outputs=3
  Demux2 : Demux  Outputs=2
  Mux : Mux  Inputs=2
  Mux1 : Mux  Inputs=3
  Selector : Selector  InputPortWidth=3  Indices=3
  Unary Minus1 : UnaryMinus
  deg2rad : Gain  Gain=pi/180  SaturateOnIntegerOverflow=on  ParamDataTypeStr=Inherit: Same as input
  ne to lat/long : Subsystem  AncestorBlock=navlibrary/ne to lat//long
  latitude mu : Outport
  longitude l : Outport  Port=2
  altitude h : Outport  Port=3
  wires:
  Demux2/1 -> latitude mu/1  "latitude"
  Demux2/2 -> longitude l/1
  Xe/1 -> Demux1/1, Selector/1
  deg2rad/1 -> Demux2/1
  ne to lat/long/1(lat_deg) -> Mux/1
  ne to lat/long/2(long_deg) -> Mux/2
  Mux/1 -> deg2rad/1
  Selector/1 -> Unary Minus1/1
  Add/1 -> altitude h/1
  altitude0/1 -> Add/2
  Mux1/1 -> ne to lat/long/1(Xe)
  Demux1/1 -> Mux1/1
  Demux1/2 -> Mux1/2
  Demux1/3 -> Mux1/3
  Unary Minus1/1 -> Add/1

== system Tricopter_Controlled/TriCopter FCS/TriCopter FCS/Build Servos PWM ==
  note: Control input
      | Rango
      | Direccion rot/Dir servos
      | Rango del servo
      |
      | eta_1 (rad) (Pan arm 1)
      | -165,165
      | -1
      | 330: -165,165
      |
      | gamma_1 (rad) (Tilt arm 1)
      | -90,15
      | -1
      | 180:-90,90 ó 330: -165,165
      |
      | eta_2 (rad) (Pan arm 2)
      | -165,165
      | -1
      | 330: -165,165
      |
      | gamma_2 (rad) (Tilt arm 2)
      | -15,90
      | 1
      | 180:-90,90
      |
      | eta_3 (rad) (Pan arm 3)
      | -165,165
      | 1
      | 330:-165,165
      |
      | gamma_3 (rad) (Tilt arm 3)
      | -90,15
      | -1
      | 180:-90,90
  signals servos in : Inport
  Demux : Demux  Outputs=6
  Mux : Mux  Inputs=6
  Signal2PWM1 : XXCopter_Control/Signal2PWM  b=deg2rad(165)  d=-deg2rad(165)  a=2100  c=900
  Signal2PWM2 : XXCopter_Control/Signal2PWM  b=deg2rad(90)  d=-deg2rad(90)  a=2100  c=900
  Signal2PWM3 : XXCopter_Control/Signal2PWM  b=deg2rad(90)  d=-deg2rad(90)  a=2100  c=900
  Signal2PWM4 : XXCopter_Control/Signal2PWM  b=deg2rad(90)  d=-deg2rad(90)  a=2100  c=900
  Signal2PWM5 : XXCopter_Control/Signal2PWM  b=deg2rad(165)  d=-deg2rad(165)  a=2100  c=900
  Signal2PWM6 : XXCopter_Control/Signal2PWM  b=deg2rad(165)  d=-deg2rad(165)  a=2100  c=900
  Unary Minus{,1..3} (4 alike) : UnaryMinus
  PWM_us servos out : Outport
  wires:
  signals servos in/1 -> Demux/1
  Demux/1 -> Unary Minus/1
  Demux/2 -> Unary Minus1/1
  Demux/3 -> Unary Minus2/1
  Demux/6 -> Unary Minus3/1
  Unary Minus3/1 -> Signal2PWM3/1
  Demux/5 -> Signal2PWM6/1
  Demux/4 -> Signal2PWM4/1
  Unary Minus2/1 -> Signal2PWM5/1
  Unary Minus1/1 -> Signal2PWM2/1
  Unary Minus/1 -> Signal2PWM1/1
  Signal2PWM1/1 -> Mux/1
  Signal2PWM2/1 -> Mux/2
  Signal2PWM5/1 -> Mux/3
  Signal2PWM4/1 -> Mux/4
  Signal2PWM6/1 -> Mux/5
  Signal2PWM3/1 -> Mux/6
  Mux/1 -> PWM_us servos out/1

== system Tricopter_Controlled/TriCopter FCS/TriCopter FCS/Control and guidance ==
  Pos_ref(m) : Inport
  Vel_ref_yaw(mps) : Inport  Port=2
  Att_ref(rad) : Inport  Port=3
  omega_b_ref : Inport  Port=4
  All_meas : Inport  Port=5
  activation_bus : Inport  Port=6
  Init_cond : Inport  Port=7
  CA_reconf : Inport  Port=8
  Enable : EnablePort  StatesWhenEnabling=reset
  Bus Selector : BusSelector  OutputSignals=Meas.Volt
  Control allocator : Subsystem  RTWFcnName=abc  RTWFileName=asas  VariantControl=Control Allocator: NO RECONFIG
      settings: MinAlgLoopOccurrences=on  RTWFcnNameOpts=User specified  RTWFileNameOpts=User specified
  Demux : Demux  Outputs=3
  Equivalent ESC signals : Product  Inputs=/*
  Equivalent Throttle : Product  Inputs=**
  Initial control deflections : Memory  X0=[throtle_1,0,0,throtle_23,eta_23,0,throtle_23,-eta_23,0]'  InheritSampleTime=on
  Inner PI Controller Quaternions : Subsystem  VariantControl=PI_quat
  NDI : Subsystem  RTWFcnName=abc  RTWFileName=asas  VariantControl=NDI: NO RECONFIG
      settings: RTWFcnNameOpts=User specified  RTWFileNameOpts=User specified
  Otter Overactuated P Controller : Subsystem  VariantControl=Overactuated P Controller
  Reference batrery level (V) : Constant  Value=16
  Safety limits : Saturate  UpperLimit=[20,20,0]'  LowerLimit=-[20,20,50]'
  Saturation1 : Saturate  UpperLimit=[10,10,v_i0]'  LowerLimit=-[10,10,2*v_i0]'
  Throttles : Selector  InputPortWidth=9  Indices=[1,4,7]
  "angles " : Selector  InputPortWidth=9  Indices=[2,3,5,6,8,9]
  keep -90/90 : Subsystem
  Mot_throtles : Outport
  Control_signals : Outport  Port=2
  Servos_angles : Outport  Port=3
  wires:
  All_meas/1 -> Otter Overactuated P Controller/3(All meas), Inner PI Controller Quaternions/6(All meas), Bus Selector/1, NDI/3(All_meas)
  NDI/3(Control_defl eval (rad)) -> Control allocator/4(Control defl prev)
  keep -90/90/1(out (rad)) -> Demux/1
  Demux/3 -> Inner PI Controller Quaternions/4(Yaw_ref (rad))
  Demux/2 -> Inner PI Controller Quaternions/3(Theta_ref (rad))
  Demux/1 -> Inner PI Controller Quaternions/2(Phi_ref (rad))
  Otter Overactuated P Controller/1(Accels des) -> Inner PI Controller Quaternions/1(Accels ref (m/s^2))
  Safety limits/1 -> Otter Overactuated P Controller/1(Position ref (m))
  Att_ref(rad)/1 -> keep -90/90/1(in (rad))
  Equivalent Throttle/1 -> Equivalent ESC signals/2
  Reference batrery level (V)/1 -> Equivalent Throttle/1
  Bus Selector/1 -> Control allocator/1(Curr_V), Equivalent ESC signals/1  "<Volt>"
  Equivalent ESC signals/1 -> Mot_throtles/1
  Control allocator/1(Control_Commands) -> "angles "/1, Control_signals/1, Throttles/1
  Throttles/1 -> Equivalent Throttle/2
  Initial control deflections/1 -> NDI/2(Control_defl for eval)
  "angles "/1 -> Servos_angles/1
  Vel_ref_yaw(mps)/1 -> Saturation1/1
  Saturation1/1 -> Otter Overactuated P Controller/2(Vel_yaw_ref(m))
  Pos_ref(m)/1 -> Safety limits/1
  Init_cond/1 -> Otter Overactuated P Controller/5(init_cond), Inner PI Controller Quaternions/8(init_cond)
  CA_reconf/1 -> Control allocator/5(CA_reconf)
  activation_bus/1 -> Otter Overactuated P Controller/4(activation_bus), Inner PI Controller Quaternions/7(activation_bus)
  Control allocator/2(Control_def for eval) -> Initial control deflections/1
  NDI/1(Virtual Control Commands) -> Control allocator/2(Forc_Mom_des)
  NDI/2(B online) -> Control allocator/3(B matrix Online)
  Inner PI Controller Quaternions/1(Accs_Ang_acc des) -> NDI/1(pseudo_control (m/s^2;rad/s^2))
  omega_b_ref/1 -> Inner PI Controller Quaternions/5(omega_b_ref_radps)

== system Tricopter_Controlled/TriCopter FCS/TriCopter FCS/Flight mode manager and commands generator ==
  Left_up : Inport
  Left_side : Inport  Port=2
  Right_up : Inport  Port=3
  Right_side : Inport  Port=4
  Safety_stab_switch : Inport  Port=5
  GCS_comm : Inport  Port=6
  All_meas : Inport  Port=7
  Bus Selector : BusSelector  OutputSignals=flight_mode_request
  Commands generator : Subsystem
  Flight manager : Subsystem
  Pos_ref(m) : Outport  PortDimensions=[3,1]
  Vel_ref_yaw(mps) : Outport  Port=2  PortDimensions=[3,1]
  Att_ref(rad) : Outport  Port=3  PortDimensions=[3,1]
  omega_b_ref : Outport  Port=4  PortDimensions=[3,1]
  flight_mode_out : Outport  Port=5
  not_allowed_transition : Outport  Port=6
  wires:
  Flight manager/1(flight_mode) -> Commands generator/1(flight_mode), flight_mode_out/1
  All_meas/1 -> Flight manager/2(All_meas), Commands generator/7(All_meas)
  Commands generator/1(Pos_ref(m)) -> Pos_ref(m)/1
  Commands generator/3(Att_ref(rad)) -> Att_ref(rad)/1
  Commands generator/2(Vel_ref_yaw(mps)) -> Vel_ref_yaw(mps)/1
  Commands generator/4(omega_b_ref) -> omega_b_ref/1
  GCS_comm/1 -> Bus Selector/1, Commands generator/6(GCS_comm)
  Bus Selector/1 -> Flight manager/1(flight_mode_request)  "<flight_mode_request>"
  Safety_stab_switch/1 -> Flight manager/3(Safety_stab_switch)
  Left_up/1 -> Commands generator/2(Left_up)
  Left_side/1 -> Commands generator/3(Left_side)
  Right_up/1 -> Commands generator/4(Right_up)
  Right_side/1 -> Commands generator/5(Right_side)
  Flight manager/2(not_allowed_transition) -> not_allowed_transition/1

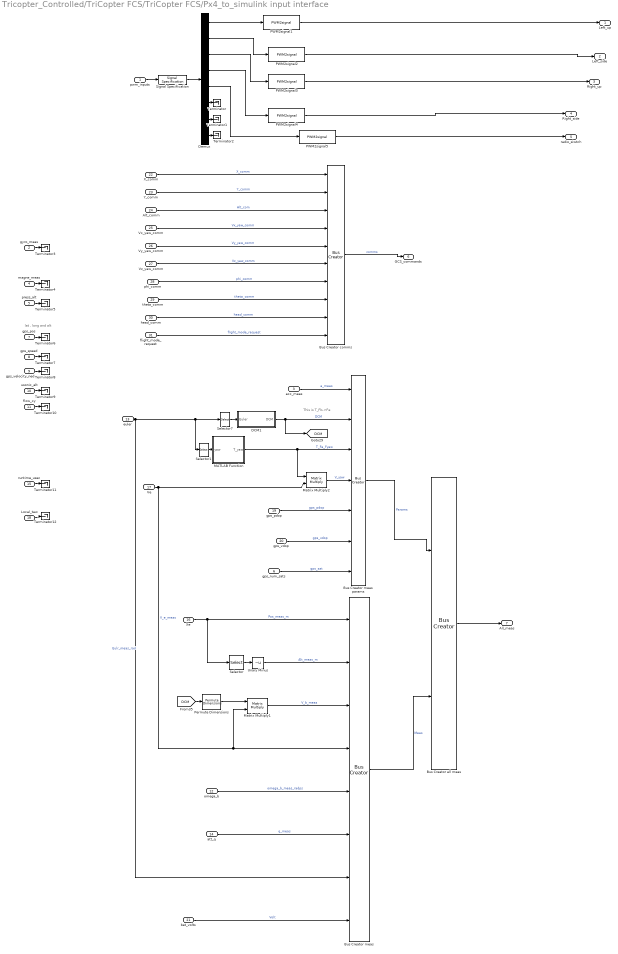
== system Tricopter_Controlled/TriCopter FCS/TriCopter FCS/Px4_to_simulink input interface ==
  note: lat , long and alt
  note: This is T_Fb->Fe
  pwm_inputs : Inport  PortDimensions=8  SampleTime=T_ctrl
  gyro_meas : Inport  Port=2  PortDimensions=3  SampleTime=T_ctrl
  acc_meas : Inport  Port=3  PortDimensions=3  SampleTime=T_ctrl
  magne_meas : Inport  Port=4  PortDimensions=3  SampleTime=T_ctrl
  press_alt : Inport  Port=5  PortDimensions=1  SampleTime=T_ctrl
  gps_num_sats : Inport  Port=6  PortDimensions=1  SampleTime=T_ctrl
  gps_pos : Inport  Port=7  PortDimensions=3  SampleTime=T_ctrl
  gps_speed : Inport  Port=8  PortDimensions=1  SampleTime=T_ctrl
  gps_velocity_ned : Inport  Port=9  PortDimensions=3  SampleTime=T_ctrl
  usonic_alt : Inport  Port=10  PortDimensions=1  SampleTime=T_ctrl
  flow_xy : Inport  Port=11  PortDimensions=2  SampleTime=T_ctrl
  omega_b : Inport  Port=12  PortDimensions=3  SampleTime=T_ctrl
  euler : Inport  Port=13  PortDimensions=3  SampleTime=T_ctrl
  att_q : Inport  Port=14  PortDimensions=4  SampleTime=T_ctrl
  runtime_usec : Inport  Port=15  PortDimensions=1  SampleTime=T_ctrl
  Xe : Inport  Port=16  PortDimensions=3  SampleTime=T_ctrl
  Ve : Inport  Port=17  PortDimensions=3  SampleTime=T_ctrl
  Local_taw : Inport  Port=18  PortDimensions=1  SampleTime=T_ctrl
  gps_pdop : Inport  Port=19  PortDimensions=1  SampleTime=T_ctrl
  gps_vdop : Inport  Port=20  PortDimensions=1  SampleTime=T_ctrl
  bat_volts : Inport  Port=21  PortDimensions=1  SampleTime=T_ctrl
  X_comm : Inport  Port=22  PortDimensions=1  SampleTime=T_ctrl
  Y_comm : Inport  Port=23  PortDimensions=1  SampleTime=T_ctrl
  Alt_comm : Inport  Port=24  PortDimensions=1  SampleTime=T_ctrl
  Vx_yaw_comm : Inport  Port=25  PortDimensions=[1,1]
  Vy_yaw_comm : Inport  Port=26  PortDimensions=1  SampleTime=T_ctrl
  Vz_yaw_comm : Inport  Port=27  PortDimensions=1  SampleTime=T_ctrl
  phi_comm : Inport  Port=28  PortDimensions=1  SampleTime=T_ctrl
  theta_comm : Inport  Port=29  PortDimensions=1  SampleTime=T_ctrl
  head_comm : Inport  Port=30  PortDimensions=1  SampleTime=T_ctrl
  flight_mode_request : Inport  Port=31  PortDimensions=1  SampleTime=T_ctrl
  Bus Creator all meas : BusCreator  Inputs=2  OutDataTypeStr=Bus: slBus2
  Bus Creator comms : BusCreator  Inputs=10  OutDataTypeStr=Bus: slBus1_comms
  Bus Creator meas : BusCreator  Inputs=8  OutDataTypeStr=Bus: Meas
  Bus Creator meas params : BusCreator  Inputs=7  OutDataTypeStr=Bus: Params
  DCM1 : Subsystem  TreatAsAtomicUnit=on
  Demux : Demux  Outputs=8
  MATLAB Function : MATLAB Function  TreatAsAtomicUnit=on
  Matrix Multiply1 : Product  Multiplication=Matrix(*)
  Matrix Multiply2 : Product  Multiplication=Matrix(*)
  PWM2signal{1..4} (4 alike) : XXCopter_Control/PWM2signal  c=1800  a=1200  d=1  b=-1
  PWM2signal5 : XXCopter_Control/PWM2signal  c=1800  a=1200  d=1  b=0
  Permute Dimensions : PermuteDimensions
  Selector : Selector  InputPortWidth=3  Indices=3
  Selector1 : Selector  InputPortWidth=3  Indices=3
  Selector7 : Selector  InputPortWidth=3  Indices=[3 2 1]
  Signal Specification : SignalSpecification  Dimensions=8
  Terminator{,1..12} (13 alike) : Terminator
  Unary Minus : UnaryMinus
  Left_up : Outport
  Left_side : Outport  Port=2
  Right_up : Outport  Port=3
  Right_side : Outport  Port=4
  radio_siwtch : Outport  Port=5
  GCS_commands : Outport  Port=6
  All_meas : Outport  Port=7
  tag scope: DCM=global
  wires:
  PWM2signal1/1 -> Left_up/1
  PWM2signal2/1 -> Left_side/1
  PWM2signal3/1 -> Right_up/1
  PWM2signal4/1 -> Right_side/1
  Bus Creator all meas/1 -> All_meas/1
  PWM2signal5/1 -> radio_siwtch/1
  Xe/1 -> Selector/1, Bus Creator meas/1  "Pos_meas_m"
  att_q/1 -> Bus Creator meas/6  "q_meas"
  Ve/1 -> Bus Creator meas/4, Matrix Multiply1/2, Matrix Multiply2/2  "V_e_meas"
  euler/1 -> Bus Creator meas/7, Selector1/1, Selector7/1  "Eulr_meas_rad"
  omega_b/1 -> Bus Creator meas/5  "omega_b_meas_radps"
  Matrix Multiply1/1 -> Bus Creator meas/3  "V_b_meas"
  Unary Minus/1 -> Bus Creator meas/2  "Alt_meas_m"
  Selector/1 -> Unary Minus/1
  bat_volts/1 -> Bus Creator meas/8  "Volt"
  Bus Creator meas/1 -> Bus Creator all meas/2  "Meas"
  Bus Creator meas params/1 -> Bus Creator all meas/1  "Params"
  DCM1/1(DCM) -> [DCM], Bus Creator meas params/2  "DCM"
  Matrix Multiply2/1 -> Bus Creator meas params/4  "V_yaw"
  acc_meas/1 -> Bus Creator meas params/1  "a_meas"
  gps_pdop/1 -> Bus Creator meas params/5  "gps_pdop"
  gps_num_sats/1 -> Bus Creator meas params/7  "gps_sat"
  gps_vdop/1 -> Bus Creator meas params/6  "gps_vdop"
  Selector7/1 -> DCM1/1(Euler)
  Selector1/1 -> MATLAB Function/1(yaw)
  MATLAB Function/1(T_yaw) -> Matrix Multiply2/1, Bus Creator meas params/3  "T_Fe_Fyaw"
  [DCM] -> Permute Dimensions/1
  Permute Dimensions/1 -> Matrix Multiply1/1
  Bus Creator comms/1 -> GCS_commands/1  "comms"
  X_comm/1 -> Bus Creator comms/1  "X_comm"
  flight_mode_request/1 -> Bus Creator comms/10  "flight_mode_request"
  Y_comm/1 -> Bus Creator comms/2  "Y_comm"
  Vx_yaw_comm/1 -> Bus Creator comms/4  "Vx_yaw_comm"
  Vy_yaw_comm/1 -> Bus Creator comms/5  "Vy_yaw_comm"
  Vz_yaw_comm/1 -> Bus Creator comms/6  "Vz_yaw_comm"
  phi_comm/1 -> Bus Creator comms/7  "phi_comm"
  theta_comm/1 -> Bus Creator comms/8  "theta_comm"
  head_comm/1 -> Bus Creator comms/9  "head_comm"
  Demux/1 -> PWM2signal1/1
  Demux/2 -> PWM2signal2/1
  Demux/3 -> PWM2signal3/1
  Demux/4 -> PWM2signal4/1
  Demux/5 -> PWM2signal5/1
  Alt_comm/1 -> Bus Creator comms/3  "Alt_com"
  pwm_inputs/1 -> Signal Specification/1
  Demux/6 -> Terminator/1
  Demux/7 -> Terminator1/1
  Demux/8 -> Terminator2/1
  gyro_meas/1 -> Terminator3/1
  magne_meas/1 -> Terminator4/1
  press_alt/1 -> Terminator5/1
  gps_pos/1 -> Terminator6/1
  gps_speed/1 -> Terminator7/1
  gps_velocity_ned/1 -> Terminator8/1
  usonic_alt/1 -> Terminator9/1
  flow_xy/1 -> Terminator10/1
  runtime_usec/1 -> Terminator11/1
  Local_taw/1 -> Terminator12/1
  Signal Specification/1 -> Demux/1
